simulink model "MPSK_passmodem"  (Simulink 9.2)
settings: Solver=FixedStepDiscrete  StartTime=0.0  StopTime=1  FixedStep=1/100000  RelTol=1e-3  AbsTol=1e-6
PreLoadFcn:
  | fs=1e5; Ts=1/fs; R=1000; T=1/R; fc=10000; M=8; offset=0;
undefined symbols (not defined in the file): gcbh, rcfiltgaincompat
libraries: commfilt2 x6, simulink_extras x2, commutil2 x2, commchan3 x1, commrandsrc2 x1
settings Model: Creator=amoura  LastModifiedBy=nox
settings SolverCC: AutoScaleAbsTol=off
settings DataIOCC: LimitDataPoints=off
settings OptimizationCC: BlockReduction=off  BooleanDataType=off  ExpressionDepthLimit=2147483647  InitFltsAndDblsToZero=on
settings DebuggingCC: SaveWithParameterizedLinksMsg=none  SignalResolutionControl=TryResolveAllWithWarning  MultiTaskDSMMsg=warning  MultiTaskCondExecSysMsg=none
settings HardwareCC: TargetUnknown=on
settings RTWCC: TemplateMakefile=grt_unix.tmf
settings GRTTargetCC: TargetFcnLib=ansi_tfl_tmw.mat  ModelReferenceCompliant=off  MatFileLogging=off

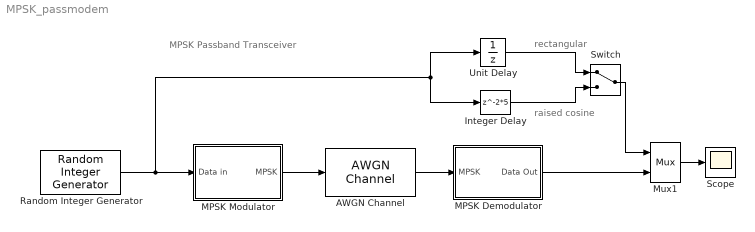
== system MPSK_passmodem ==
  note: raised cosine
  note: rectangular
  note: MPSK Passband Transceiver
  AWGN Channel : commchan3/AWGN Channel  InputProcessing=Columns as channels (frame based)  seed=67  noiseMode="Signal to noise ratio  (Es/No)"  EbNodB=0  EsNodB=100  SNRdB=10  bitsPerSym=1  Ps=1  Tsym=T  variance=0.1
  Integer Delay : Delay  DelayLength=2*5  InitialCondition=0
  MPSK Demodulator : Subsystem
  MPSK Modulator : Subsystem
  Mux1 : Mux  Inputs=2
  Random Integer Generator : commrandsrc2/Random Integer Generator  mul=M  seed=96931  Ts=T  frameBased=off  sampPerFrame=100  orient=off  outDataType=double
  Scope : Scope
  Switch : ManualSwitch
  Unit Delay : UnitDelay  SampleTime=T
  wires:
  MPSK Modulator/1(MPSK) -> AWGN Channel/1
  Mux1/1 -> Scope/1
  Random Integer Generator/1 -> MPSK Modulator/1(Data in), Unit Delay/1, Integer Delay/1
  MPSK Demodulator/1(Data Out) -> Mux1/2
  AWGN Channel/1 -> MPSK Demodulator/1(MPSK)
  Integer Delay/1 -> Switch/2
  Unit Delay/1 -> Switch/1
  Switch/1 -> Mux1/1

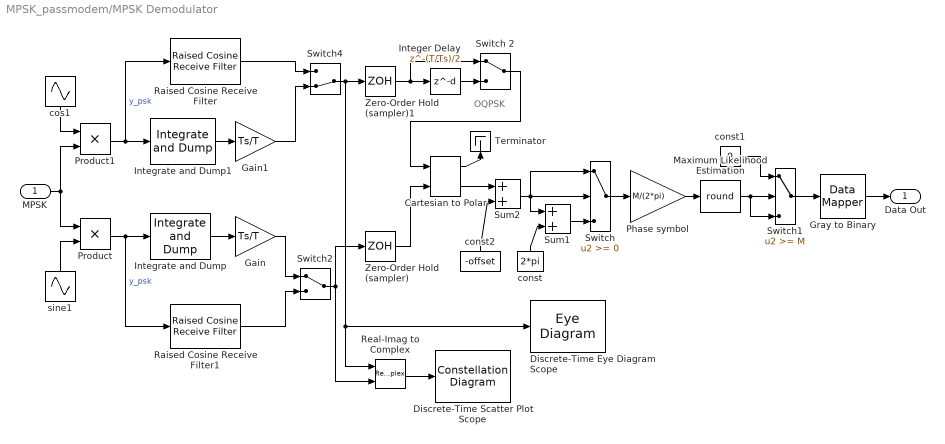
== system MPSK_passmodem/MPSK Demodulator ==
  note: OQPSK
  MPSK : Inport
  Cartesian to Polar : simulink_extras/Transformations/Cartesian to Polar
      settings: SourceProductName=Simulink
  Discrete-Time Eye Diagram Scope : EyeDiagram  Tag=EyeDiagram
  Discrete-Time Scatter Plot Scope : ConstellationDiagram  Tag=ScatterPlot
  Gain : Gain  Gain=Ts/T  SampleTime=Ts  SaturateOnIntegerOverflow=on  OutDataTypeStr=Inherit: Same as input  ParamDataTypeStr=Inherit: Same as input
  Gain1 : Gain  Gain=Ts/T  SampleTime=Ts  SaturateOnIntegerOverflow=on  OutDataTypeStr=Inherit: Same as input  ParamDataTypeStr=Inherit: Same as input
  Gray to Binary : commutil2/Data Mapper  MapMode=Gray to Binary  M=M  MapVec=[0 1 3 2 7 6 4 5]
      settings: SourceProductName=Communications System Toolbox  SourceProductBaseCode=CM
  Integer Delay : Delay  DelayLength=(T/Ts)/2  InitialCondition=0
  Integrate and Dump : commfilt2/Integrate and Dump  obssamples=T/Ts  offsetsamples=1  nodump=on  roundingMode=Floor  overflowMode=off  outputDataTypeStr=Inherit: Same as accumulator  outputLastDataTypeStr=Inherit: Same as accumulator
      settings: SourceProductName=Communications System Toolbox
  Integrate and Dump1 : commfilt2/Integrate and Dump  obssamples=T/Ts  offsetsamples=1  nodump=on  roundingMode=Floor  overflowMode=off  outputDataTypeStr=Inherit: Same as accumulator  outputLastDataTypeStr=Inherit: Same as accumulator
      settings: SourceProductName=Communications System Toolbox
  Maximum Likelihood Estimation : Rounding  Operator=round
  Phase symbol : Gain  Gain=M/(2*pi)  SaturateOnIntegerOverflow=on  OutDataTypeStr=Inherit: Same as input  ParamDataTypeStr=Inherit: Same as input
  Product : Product  SampleTime=1/100000  SaturateOnIntegerOverflow=on  RndMeth=Zero  InputSameDT=on  OutDataTypeStr=Inherit: Same as first input
  Product1 : Product  SampleTime=1/100000  SaturateOnIntegerOverflow=on  RndMeth=Zero  InputSameDT=on  OutDataTypeStr=Inherit: Same as first input
  Raised Cosine Receive Filter : commfilt2/Raised Cosine Receive Filter  filtType=Square root  R=0.4  filtSpan=2*(5)  N=100  downFactor=1  downOffset=0  filterGain=rcfiltgaincompat(gcbh)  InputProcessing=Columns as channels (frame based)  RateOptions=Enforce single-rate processing  framing=Mute  checkCoeff=off  variableName=rcRxFilt  currentFiltSpan=2*(5)  D=5  inputOffset=0  sampMode=Mute  saveAsFlag=0  rateMode=Downsampling  checkGain=Normalized  launchFVT=off  roundingMode=Floor  overflowMode=off  coeffDataTypeStr=Inherit: Same word length as input  coeffMin=[]  coeffMax=[]  coeffLastDataTypeStr=Inherit: Same word length as input  accumDataTypeStr=Inherit: Same as product output  accumLastDataTypeStr=Inherit: Same as product output  outputDataTypeStr=Inherit: Same as accumulator  outputMin=[]  outputMax=[]  outputLastDataTypeStr=Inherit: Same as accumulator
  Raised Cosine Receive Filter1 : commfilt2/Raised Cosine Receive Filter  filtType=Square root  R=0.4  filtSpan=2*(5)  N=100  downFactor=1  downOffset=0  filterGain=rcfiltgaincompat(gcbh)  InputProcessing=Columns as channels (frame based)  RateOptions=Enforce single-rate processing  framing=Mute  checkCoeff=off  variableName=rcRxFilt1  currentFiltSpan=2*(5)  D=5  inputOffset=0  sampMode=Mute  saveAsFlag=0  rateMode=Downsampling  checkGain=Normalized  launchFVT=off  roundingMode=Floor  overflowMode=off  coeffDataTypeStr=Inherit: Same word length as input  coeffMin=[]  coeffMax=[]  coeffLastDataTypeStr=Inherit: Same word length as input  accumDataTypeStr=Inherit: Same as product output  accumLastDataTypeStr=Inherit: Same as product output  outputDataTypeStr=Inherit: Same as accumulator  outputMin=[]  outputMax=[]  outputLastDataTypeStr=Inherit: Same as accumulator
  Real-Imag to Complex : RealImagToComplex
  Sum1 : Sum  SaturateOnIntegerOverflow=on  InputSameDT=on  OutDataTypeStr=Inherit: Same as first input
  Sum2 : Sum  SaturateOnIntegerOverflow=on  InputSameDT=on  OutDataTypeStr=Inherit: Same as first input
  Switch : Switch  SaturateOnIntegerOverflow=on  InputSameDT=on
  Switch 2 : ManualSwitch
  Switch1 : Switch  Threshold=M
  Switch2 : ManualSwitch
  Switch4 : ManualSwitch  CurrentSetting=0
  Terminator : Terminator
  Zero-Order Hold (sampler) : ZeroOrderHold  SampleTime=T
  Zero-Order Hold (sampler)1 : ZeroOrderHold  SampleTime=T
  const : Constant  Value=2*pi
  const1 : Constant  Value=0
  const2 : Constant  Value=-offset
  cos1 : Sin  Frequency=2*pi*fc  Phase=pi/2  SampleTime=0
  sine1 : Sin  Frequency=2*pi*fc  SampleTime=0
  Data Out : Outport
  wires:
  Product/1 -> Raised Cosine Receive Filter1/1, Integrate and Dump/1  "y_psk"
  MPSK/1 -> Product1/2, Product/1
  Integrate and Dump/1 -> Gain/1
  sine1/1 -> Product/2
  Product1/1 -> Integrate and Dump1/1, Raised Cosine Receive Filter/1  "y_psk"
  Integrate and Dump1/1 -> Gain1/1
  cos1/1 -> Product1/1
  Sum1/1 -> Switch/3
  Switch/1 -> Phase symbol/1
  Cartesian to Polar/1 -> Terminator/1
  Phase symbol/1 -> Maximum Likelihood Estimation/1
  Zero-Order Hold (sampler)/1 -> Cartesian to Polar/2
  const/1 -> Sum1/2
  Switch1/1 -> Gray to Binary/1
  Maximum Likelihood Estimation/1 -> Switch1/2, Switch1/3
  const1/1 -> Switch1/1
  Real-Imag to Complex/1 -> Discrete-Time Scatter Plot Scope/1
  Gray to Binary/1 -> Data Out/1
  Sum2/1 -> Switch/1, Sum1/1, Switch/2
  Raised Cosine Receive Filter/1 -> Switch4/1
  Gain1/1 -> Switch4/2
  Switch4/1 -> Zero-Order Hold (sampler)1/1, Discrete-Time Eye Diagram Scope/1, Real-Imag to Complex/1
  Gain/1 -> Switch2/1
  Switch2/1 -> Zero-Order Hold (sampler)/1, Real-Imag to Complex/2
  const2/1 -> Sum2/2
  Cartesian to Polar/2 -> Sum2/1
  Raised Cosine Receive Filter1/1 -> Switch2/2
  Integer Delay/1 -> Switch 2/2
  Zero-Order Hold (sampler)1/1 -> Integer Delay/1, Switch 2/1
  Switch 2/1 -> Cartesian to Polar/1

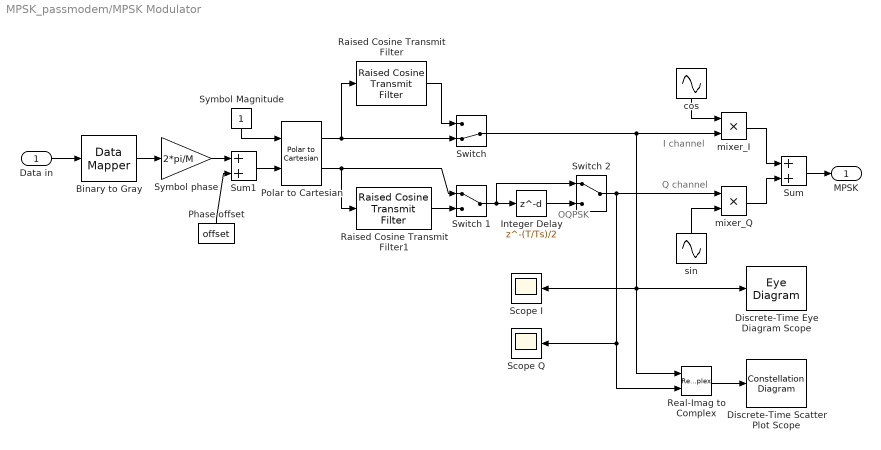
== system MPSK_passmodem/MPSK Modulator ==
  note: I channel
  note: Q channel
  note: OQPSK
  Data in : Inport
  Binary to Gray : commutil2/Data Mapper  MapMode=Binary to Gray  M=M  MapVec=[0 1 3 2 7 6 4 5]
      settings: SourceProductName=Communications System Toolbox  SourceProductBaseCode=CM
  Discrete-Time Eye Diagram Scope : EyeDiagram  Tag=EyeDiagram
  Discrete-Time Scatter Plot Scope : ConstellationDiagram  Tag=ScatterPlot
  Integer Delay : Delay  DelayLength=(T/Ts)/2  InitialCondition=0
  Phase offset : Constant  Value=offset  SampleTime=T
  Polar to Cartesian : simulink_extras/Transformations/Polar to Cartesian
      settings: SourceProductName=Simulink  SourceProductBaseCode=SL
  Raised Cosine Transmit Filter : commfilt2/Raised Cosine Transmit Filter  filtType=Square root  R=0.4  filtSpan=2*(5)  N=100  filterGain=rcfiltgaincompat(gcbh)  RateOptions=Allow multirate processing  framing=Mute  checkCoeff=off  variableName=rcTxFilt  checkGain=Normalized  sampMode=Mute  saveAsFlag=0  currentFiltSpan=2*(5)  D=5  launchFVT=off  roundingMode=Floor  overflowMode=off  coeffDataTypeStr=Inherit: Same word length as input  coeffMin=[]  coeffMax=[]  coeffLastDataTypeStr=Inherit: Same word length as input  outputDataTypeStr=Inherit: Same as accumulator  outputMin=[]  outputMax=[]  outputLastDataTypeStr=Inherit: Same as accumulator
  Raised Cosine Transmit Filter1 : commfilt2/Raised Cosine Transmit Filter  filtType=Square root  R=0.4  filtSpan=2*(5)  N=100  filterGain=rcfiltgaincompat(gcbh)  RateOptions=Allow multirate processing  framing=Mute  checkCoeff=off  variableName=rcTxFilt1  checkGain=Normalized  sampMode=Mute  saveAsFlag=0  currentFiltSpan=2*(5)  D=5  launchFVT=off  roundingMode=Floor  overflowMode=off  coeffDataTypeStr=Inherit: Same word length as input  coeffMin=[]  coeffMax=[]  coeffLastDataTypeStr=Inherit: Same word length as input  outputDataTypeStr=Inherit: Same as accumulator  outputMin=[]  outputMax=[]  outputLastDataTypeStr=Inherit: Same as accumulator
  Real-Imag to Complex : RealImagToComplex
  Scope I : Scope
  Scope Q : Scope
  Sum : Sum  SaturateOnIntegerOverflow=on  InputSameDT=on  OutDataTypeStr=Inherit: Same as first input
  Sum1 : Sum  SaturateOnIntegerOverflow=on  InputSameDT=on  OutDataTypeStr=Inherit: Same as first input
  Switch : ManualSwitch  CurrentSetting=0
  Switch 1 : ManualSwitch
  Switch 2 : ManualSwitch
  Symbol Magnitude : Constant  SampleTime=T
  Symbol phase : Gain  Gain=2*pi/M  SaturateOnIntegerOverflow=on  OutDataTypeStr=Inherit: Same as input  ParamDataTypeStr=Inherit: Same as input
  cos : Sin  Frequency=2*pi*fc  Phase=pi/2  SampleTime=0
  mixer_I : Product  SampleTime=Ts  SaturateOnIntegerOverflow=on  InputSameDT=on  OutDataTypeStr=Inherit: Same as first input
  mixer_Q : Product  SampleTime=Ts  SaturateOnIntegerOverflow=on  InputSameDT=on  OutDataTypeStr=Inherit: Same as first input
  sin : Sin  Frequency=2*pi*fc  SampleTime=0
  MPSK : Outport
  wires:
  Symbol Magnitude/1 -> Polar to Cartesian/1
  mixer_I/1 -> Sum/1
  mixer_Q/1 -> Sum/2
  sin/1 -> mixer_Q/2
  Binary to Gray/1 -> Symbol phase/1
  Sum/1 -> MPSK/1
  Data in/1 -> Binary to Gray/1
  Polar to Cartesian/1 -> Raised Cosine Transmit Filter/1, Switch/2
  Polar to Cartesian/2 -> Raised Cosine Transmit Filter1/1, Switch 1/1
  cos/1 -> mixer_I/1
  Symbol phase/1 -> Sum1/1
  Phase offset/1 -> Sum1/2
  Sum1/1 -> Polar to Cartesian/2
  Raised Cosine Transmit Filter/1 -> Switch/1
  Switch/1 -> mixer_I/2, Scope I/1, Discrete-Time Eye Diagram Scope/1, Real-Imag to Complex/1
  Raised Cosine Transmit Filter1/1 -> Switch 1/2
  Switch 1/1 -> Switch 2/1, Integer Delay/1
  Integer Delay/1 -> Switch 2/2
  Switch 2/1 -> mixer_Q/1, Scope Q/1, Real-Imag to Complex/2
  Real-Imag to Complex/1 -> Discrete-Time Scatter Plot Scope/1
